simulink model "DiagramaBloque"  (Simulink 7.9)
settings: Solver=ode45  StartTime=0.0  StopTime=300  RelTol=1e-3
settings Model: Creator=soto  LastModifiedBy=Usuario

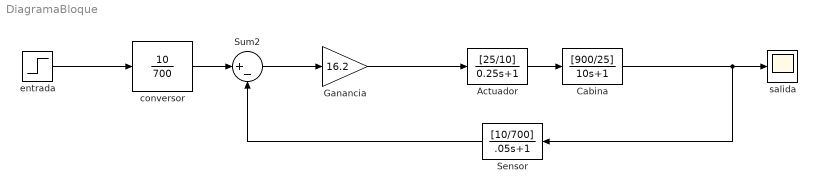
== system DiagramaBloque ==
  Actuador : TransferFcn  Numerator=[25/10]  Denominator=[0.25 1]
  Cabina : TransferFcn  Numerator=[900/25]  Denominator=[10 1]
  Ganancia : Gain  Gain=16.2
  Sensor : TransferFcn  Numerator=[10/700]  Denominator=[.05 1]
  Sum2 : Sum  Inputs=|+-
  conversor : TransferFcn  Numerator=[0 0 10]  Denominator=[0 0 700]
  "entrada " : Step  Time=0  After=700  SampleTime=1
  salida : Scope
      settings: TimeRange=2.560000000000001  YMin=0  YMax=500
  wires:
  conversor/1 -> Sum2/1
  Cabina/1 -> salida/1, Sensor/1
  Actuador/1 -> Cabina/1
  "entrada "/1 -> conversor/1
  Sensor/1 -> Sum2/2
  Sum2/1 -> Ganancia/1
  Ganancia/1 -> Actuador/1
